simulink library "ddm"  (R2021b)
settings: Solver=VariableStepAuto  StartTime=0.0  StopTime=10.0  RelTol=1e-3
undefined symbols (not defined in the file or in its folder): ENUM_ADASACCSTA_ERROR, ENUM_ADASACCSTA_OFF, ENUM_ADASACCSTA_STANDBY, ENUM_ADASISASTA_OFF, ENUM_ALLOWMOV_ALLOWREADY, ENUM_APS, ENUM_BRKSTA_ERROR, ENUM_BRKSTA_OFF, ENUM_BRKSTA_ON, ENUM_BRKSW_INVALID, ENUM_BRKSW_OFF, ENUM_BRKSW_ON, ENUM_CHGPREACTERRSTA_OBCPRE, ENUM_DCDCFAULTSTA_ANYFAULTLV1, ENUM_DCDCFAULTSTA_ANYFAULTLV2, ENUM_DRIVETRAIN_AWD, ENUM_DRIVETRAIN_FWD, ENUM_DRIVETRAIN_RWD, ENUM_DRSEATSTA_INVALID, ENUM_EDUDRTSTA_NORMAL, ENUM_EPBSTA_APPLIED, ENUM_EPBSTA_RELEASED, ENUM_HVBATTREADYPRE_READY, ENUM_MCUWARN_LV0, ENUM_MCUWARN_LV1, ENUM_MCUWARN_LV2, ENUM_MCUWARN_LV3, ENUM_MCUWARN_NOERROR, ENUM_OBCFAULTSTA_ANYFAULT, ENUM_PAS_R2F2, ENUM_PDFAULT_BATTPDFAIL, ENUM_PDFAULT_DCDCDISABLE, ENUM_PDFAULT_MCUDISABLE, ENUM_PDFAULT_MCUDISCHRG, ENUM_POWERSTA_OFF, ENUM_POWERSTA_ON, ENUM_POWERSTA_READY, ENUM_POWERSTA_STANDBY, ENUM_PRESSINDI_LOW, ENUM_PUFAULT_BATTUPFAIL, ENUM_PUFAULT_DCDCENABLEFAIL, ENUM_PUFAULT_PRECHRGCHKFAIL, ENUM_PUFAULT_SAFETYCHKFAIL, ENUM_PUSTATE_COMPLETED, ENUM_PWRSTASW_OFF, ENUM_PWRSTASW_OFFA, ENUM_PWRSTASW_OFFCHVCHRG, ENUM_PWRSTASW_OFFCLVCHRG, ENUM_PWRSTASW_ON, ENUM_PWRSTASW_ONHVCHRG, ENUM_PWRSTASW_READY, ENUM_PWRSTASW_STANDBY, ENUM_RANGESTA_12IN, ENUM_SHIFTCOMMAND_D, ENUM_SHIFTCOMMAND_N, ENUM_SHIFTCOMMAND_P, ENUM_SHIFTCOMMAND_R, ENUM_VEHMALFUNLV_2ND, ENUM_VEHMALFUNLV_3RD, ENUM_VEHMALFUNLV_4TH ... (+835)
libraries: hcu_lib x750, $bdroot x12, simulink x5
(part 4 of 28)

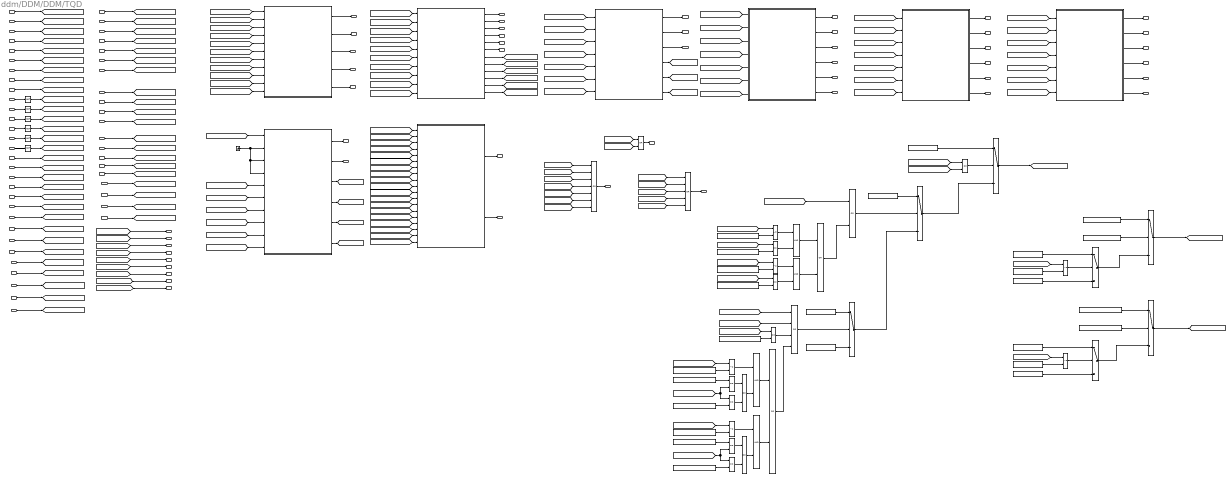
== system ddm/DDM/DDM/TQD ==
  VPMM_SysPwrSta_enum : Inport
  VINP_AccelPedal1Vol_V : Inport  Port=2
  VINP_AccelPedal2Vol_V : Inport  Port=3
  VDHP_EAPS12RangeSta_enum : Inport  Port=4
  VDHP_EAPCRBAD_flg : Inport  Port=5
  task_time_s : Inport  Port=6
  DTC_clear_request : Inport  Port=7
  No_CAN3_BUS_OFF : Inport  Port=8
  No_CAN1_BUS_OFF : Inport  Port=9
  VINP_CANMsgValidMCUF1_flg : Inport  Port=10
  VINP_CANMsgValidMCUR1_flg : Inport  Port=11
  VINP_CANMsgValidShifter1_flg : Inport  Port=12
  VINP_CANMsgValidESC7_flg : Inport  Port=13
  VINP_CANMsgValidESC1_flg : Inport  Port=14
  VINP_CANMsgValidESC5_flg : Inport  Port=15
  VDDM_MCUF1RCErr_flg : Inport  Port=16
  VDDM_MCUF1CSErr_flg : Inport  Port=17
  VDDM_MCUR1RCErr_flg : Inport  Port=18
  VDDM_MCUR1CSErr_flg : Inport  Port=19
  VDDM_Shifter1RCErr_flg : Inport  Port=20
  VDDM_Shifter1CSErr_flg : Inport  Port=21
  VDDM_ESC7RCErr_flg : Inport  Port=22
  VDDM_ESC7CSErr_flg : Inport  Port=23
  VDDM_ESC1RCErr_flg : Inport  Port=24
  VDDM_ESC1CSErr_flg : Inport  Port=25
  VDDM_ESC5RCErr_flg : Inport  Port=26
  VDDM_ESC5CSErr_flg : Inport  Port=27
  VINP_FrEDUDrtSta_flg : Inport  Port=28
  VINP_VehSpeed_kph : Inport  Port=29
  VINP_FrEDURealTMTq_Nm : Inport  Port=30
  VTQR_FrTMTqReq_Nm : Inport  Port=31
  VINP_RrEDUDrtSta_flg : Inport  Port=32
  VINP_RrEDURealTMTq_Nm : Inport  Port=33
  VTQR_RrTMTqReq_Nm : Inport  Port=34
  VINP_MCUWarnF_enum : Inport  Port=35
  VINP_MCUWarnR_enum : Inport  Port=36
  VINP_Pedal1Ref5V_V : Inport  Port=37
  VINP_Pedal2Ref5V_V : Inport  Port=38
  VINP_HVBattSOC_pct : Inport  Port=39
  VDDM_AuxBattVolV_V : Inport  Port=40
  VTQD_ActParkRequest_flg : Inport  Port=41
  VINP_EPBSta_enum : Inport  Port=42
  VINP_ShifterHandleCmd_enum : Inport  Port=43
  VINP_BMSWarn4_flg : Inport  Port=44
  VINP_BMSWarn5_flg : Inport  Port=45
  VINP_BMSWarn6_flg : Inport  Port=46
  VINP_BMSWarn7_flg : Inport  Port=47
  VINP_BMSWarn8_flg : Inport  Port=48
  VINP_DCDCFaultSta_enum : Inport  Port=49
  VPMM_DrivetrainSelect_enum : Inport  Port=50
  APS_DDM : Subsystem
  Constant1 : Constant  Value=ENUM_DRIVETRAIN_FWD
  Constant10 : Constant  Value=ENUM_MCUWARN_LV3
  Constant11 : Constant  Value=ENUM_VEHMALFUNLV_3RD
  Constant12 : Constant  Value=ENUM_VEHMALFUNLV_4TH
  Constant13 : Constant  Value=KDDM_LimpHomeActTmp_flg_ovrdflg  OutDataTypeStr=Inherit: Inherit via back propagation
  Constant14 : Constant  Value=KDDM_LimpHomeActTmp_flg_ovrdval  OutDataTypeStr=Inherit: Inherit via back propagation
  Constant15 : Constant  Value=ENUM_VEHMALFUNLV_2ND
  Constant16 : Constant  Value=ENUM_VEHMALFUNLV_NORMAL
  Constant17 : Constant  Value=ENUM_DCDCFAULTSTA_ANYFAULTLV2
  Constant18 : Constant  Value=ENUM_VEHMALFUNLV_2ND
  Constant19 : Constant  Value=TRUE
  Constant2 : Constant  Value=ENUM_MCUWARN_LV1
  Constant20 : Constant  Value=FALSE
  Constant21 : Constant  Value=ENUM_VEHMALFUNLV_3RD
  Constant22 : Constant  Value=TRUE
  Constant23 : Constant  Value=FALSE
  Constant24 : Constant  Value=KDDM_EDriveSysErrVCUTmp_ovrdflg  OutDataTypeStr=Inherit: Inherit via back propagation
  Constant25 : Constant  Value=KDDM_EDriveSysErrVCUTmp_ovrdval  OutDataTypeStr=Inherit: Inherit via back propagation
  Constant3 : Constant  Value=ENUM_MCUWARN_LV2
  Constant4 : Constant  Value=ENUM_DRIVETRAIN_RWD
  Constant5 : Constant  Value=ENUM_MCUWARN_LV1
  Constant6 : Constant  Value=ENUM_MCUWARN_LV2
  Constant7 : Constant  Value=ENUM_DRIVETRAIN_FWD
  Constant8 : Constant  Value=ENUM_DRIVETRAIN_RWD
  Constant9 : Constant  Value=ENUM_MCUWARN_LV3
  EPB : Subsystem
  ESC1_DDM : Subsystem
  ESC5_DDM : Subsystem
  ESC7_DDM : Subsystem
  Equal{1,5,8,11} (4 alike) : RelationalOperator  Operator=~=  OutDataTypeStr=boolean  RndMeth=Simplest
  Equal{2..4,6..7,9..10} (7 alike) : RelationalOperator  Operator===  OutDataTypeStr=boolean  RndMeth=Simplest
  Equal12 : RelationalOperator  OutDataTypeStr=boolean  RndMeth=Simplest
  Equal13 : RelationalOperator  OutDataTypeStr=boolean  RndMeth=Simplest
  Ground : Ground
  Logical Operator{,1..5} (6 alike) : Logic  Operator=NOT  AllPortsSameDT=off  OutDataTypeStr=boolean
  MCU1_DDM : Subsystem
  MCU_DDM : Subsystem
  OR : Logic  Operator=OR  Inputs=5  AllPortsSameDT=off  OutDataTypeStr=boolean
  OR1 : Logic  Operator=OR  Inputs=7  AllPortsSameDT=off  OutDataTypeStr=boolean
  OR{2,4,6..7,9..10,12} (7 alike) : Logic  Operator=OR  AllPortsSameDT=off  OutDataTypeStr=boolean
  OR{5,8,11,13} (4 alike) : Logic  AllPortsSameDT=off  OutDataTypeStr=boolean
  OR3 : Logic  Operator=OR  Inputs=4  AllPortsSameDT=off  OutDataTypeStr=boolean
  Shifter1_DDM : Subsystem
  Switch{1..7} (7 alike) : Switch  Criteria=u2 ~= 0
  VDDM_APS1SigOoRDTC_raw32 : Outport
  VDDM_APS2SigOoRDTC_raw32 : Outport  Port=2
  VDDM_APSCorrErrDTC_raw32 : Outport  Port=3
  VDDM_MCUF1NoComDTC_raw32 : Outport  Port=4
  VDDM_MCUR1NoComDTC_raw32 : Outport  Port=5
  VDDM_Shifter1NoComDTC_raw32 : Outport  Port=6
  VDDM_ESC7NoComDTC_raw32 : Outport  Port=7
  VDDM_ESC1NoComDTC_raw32 : Outport  Port=8
  VDDM_ESC5NoComDTC_raw32 : Outport  Port=9
  VDDM_MCUF1RCErrDTC_raw32 : Outport  Port=10
  VDDM_MCUR1RCErrDTC_raw32 : Outport  Port=11
  VDDM_MCUF1CSErrDTC_raw32 : Outport  Port=12
  VDDM_MCUR1CSErrDTC_raw32 : Outport  Port=13
  VDDM_Shifter1RCErrDTC_raw32 : Outport  Port=14
  VDDM_Shifter1CSErrDTC_raw32 : Outport  Port=15
  VDDM_ESC7RCErrDTC_raw32 : Outport  Port=16
  VDDM_ESC7CSErrDTC_raw32 : Outport  Port=17
  VDDM_ESC1RCErrDTC_raw32 : Outport  Port=18
  VDDM_ESC1CSErrDTC_raw32 : Outport  Port=19
  VDDM_ESC5RCErrDTC_raw32 : Outport  Port=20
  VDDM_ESC5CSErrDTC_raw32 : Outport  Port=21
  VDDM_FrMCUTqErrDTC_raw32 : Outport  Port=22
  VDDM_RrMCUTqErrDTC_raw32 : Outport  Port=23
  VDDM_MCUF1NoComCFS_flg : Outport  Port=24
  VDDM_MCUF1RCErrCFS_flg : Outport  Port=25
  VDDM_MCUF1CSErrCFS_flg : Outport  Port=26
  VDDM_MCUR1NoComCFS_flg : Outport  Port=27
  VDDM_MCUR1RCErrCFS_flg : Outport  Port=28
  VDDM_MCUR1CSErrCFS_flg : Outport  Port=29
  VDDM_ESC7NoComCFS_flg : Outport  Port=30
  VDDM_ESC7RCErrCFS_flg : Outport  Port=31
  VDDM_ESC7CSErrCFS_flg : Outport  Port=32
  VDDM_ESC1NoComCFS_flg : Outport  Port=33
  VDDM_ESC1RCErrCFS_flg : Outport  Port=34
  VDDM_ESC1CSErrCFS_flg : Outport  Port=35
  VDDM_ESC5NoComCFS_flg : Outport  Port=36
  VDDM_ESC5RCErrCFS_flg : Outport  Port=37
  VDDM_ESC5CSErrCFS_flg : Outport  Port=38
  VDDM_5vAPS1PwrErrDTC_raw32 : Outport  Port=39
  VDDM_5vAPS2PwrErrDTC_raw32 : Outport  Port=40
  VDDM_EPBLockTODTC_raw32 : Outport  Port=41
  VDDM_EPBUnlockTODTC_raw32 : Outport  Port=42
  EDriveSysErr_VCUErr : Outport  Port=43
  EDriveSysErr_ShifterErr : Outport  Port=44
  EngageP_Fail : Outport  Port=45
  VDDM_LimpHomeActTmp_flg : Outport  Port=46
  VDDM_EDriveSysErr_VCUErrTmp_flg : Outport  Port=47
  VDDM_VehMalfunLevelTmp_enum : Outport  Port=48
  wires:
  VINP_ShifterHandleCmd_enum/1 -> [VINP_ShifterHandleCmd_enum]
  VINP_EPBSta_enum/1 -> [VINP_EPBSta_enum]
  VTQD_ActParkRequest_flg/1 -> [VTQD_ActParkRequest_flg]
  EPB/2(VDDM_EPBUnlockTODTC_raw32) -> VDDM_EPBUnlockTODTC_raw32/1
  EPB/1(VDDM_EPBLockTODTC_raw32) -> VDDM_EPBLockTODTC_raw32/1
  [VINP_EPBSta_enum] -> EPB/7(VINP_EPBSta_enum)
  [VTQD_ActParkRequest_flg] -> EPB/6(VTQD_ActParkRequest_flg)
  [VINP_ShifterHandleCmd_enum] -> EPB/8(VINP_ShifterHandleCmd_enum)
  [VPMM_SysPwrSta_enum] -> EPB/5(VPMM_SysPwrSta_enum)
  [task_time_s] -> EPB/9(task_time_s)
  [No_CAN1_BUS_OFF] -> EPB/1(NO_CAN1_BUS_OFF)
  [DTC_clear_request] -> EPB/10(DTC_clear_request)
  Ground/1 -> EPB/2(CAN_LossOfEPB1), EPB/3(RC_LossErrOfEPB1), EPB/4(CS_LossErrOfEPB1)
  [VDDM_AuxBattVolV_V] -> APS_DDM/11(VDDM_AuxBattVolV_V)
  VDDM_AuxBattVolV_V/1 -> [VDDM_AuxBattVolV_V]
  APS_DDM/5(VDDM_5vAPS2PwrErrDTC_raw32) -> VDDM_5vAPS2PwrErrDTC_raw32/1
  APS_DDM/4(VDDM_5vAPS1PwrErrDTC_raw32) -> VDDM_5vAPS1PwrErrDTC_raw32/1
  [VINP_HVBattSOC_pct] -> APS_DDM/8(VINP_HVBattSOC_pct)
  VINP_HVBattSOC_pct/1 -> [VINP_HVBattSOC_pct]
  [VINP_Pedal2Ref5V_V] -> APS_DDM/7(VINP_Pedal2Ref5V_V)
  [VINP_Pedal1Ref5V_V] -> APS_DDM/6(VINP_Pedal1Ref5V_V)
  VINP_Pedal2Ref5V_V/1 -> [VINP_Pedal2Ref5V_V]
  VINP_Pedal1Ref5V_V/1 -> [VINP_Pedal1Ref5V_V]
  [VDDM_MCUR1RCErrCFS_flg] -> MCU_DDM/12(VDDM_MCUR1RCErrCFS_flg)
  [VDDM_MCUF1RCErrCFS_flg] -> MCU_DDM/5(VDDM_MCUF1RCErrCFS_flg)
  [VDDM_MCUF1CSErrCFS_flg] -> MCU_DDM/6(VDDM_MCUF1CSErrCFS_flg)
  [No_CAN3_BUS_OFF] -> MCU_DDM/3(No_CAN3_BUS_OFF)
  [VINP_MCUWarnF_enum] -> MCU_DDM/17(VINP_MCUWarnF_enum)
  [VINP_RrEDUDrtSta_flg] -> MCU_DDM/14(VINP_RrEDUDrtSta_flg)
  [VDDM_MCUR1CSErrCFS_flg] -> MCU_DDM/13(VDDM_MCUR1CSErrCFS_flg)
  [VPMM_SysPwrSta_enum] -> MCU_DDM/2(VPMM_SysPwrSta_enum)
  [VDDM_MCUF1NoComCFS_flg] -> MCU_DDM/4(VDDM_MCUF1NoComCFS_flg)
  [VTQR_FrTMTqReq_Nm] -> MCU_DDM/10(VTQR_FrTMTqReq_Nm)
  [task_time_s] -> MCU_DDM/1(task_time_s)
  [VTQR_RrTMTqReq_Nm] -> MCU_DDM/16(VTQR_RrTMTqReq_Nm)
  [VINP_FrEDUDrtSta_flg] -> MCU_DDM/8(VINP_FrEDUDrtSta_flg)
  [VINP_FrEDURealTMTq_Nm] -> MCU_DDM/9(VINP_FrEDURealTMTq_Nm)
  [VINP_RrEDURealTMTq_Nm] -> MCU_DDM/15(VINP_RrEDURealTMTq_Nm)
  [DTC_clear_request] -> MCU_DDM/19(DTC_clear_request)
  [VDDM_MCUR1NoComCFS_flg] -> MCU_DDM/11(VDDM_MCUR1NoComCFS_flg)
  [VINP_MCUWarnR_enum] -> MCU_DDM/18(VINP_MCUWarnR_enum)
  [VINP_VehSpeed_kph] -> MCU_DDM/7(VINP_VehSpeed_kph)
  [VDDM_MCUF1RCErrCFS_flg] -> VDDM_MCUF1RCErrCFS_flg/1
  [VDDM_MCUR1RCErrCFS_flg] -> VDDM_MCUR1RCErrCFS_flg/1
  [VDDM_MCUR1NoComCFS_flg] -> VDDM_MCUR1NoComCFS_flg/1
  [VDDM_MCUF1CSErrCFS_flg] -> VDDM_MCUF1CSErrCFS_flg/1
  [VDDM_MCUR1CSErrCFS_flg] -> VDDM_MCUR1CSErrCFS_flg/1
  [VDDM_MCUF1NoComCFS_flg] -> VDDM_MCUF1NoComCFS_flg/1
  MCU1_DDM/11(VDDM_MCUR1RCErrCFS_flg) -> [VDDM_MCUR1RCErrCFS_flg]
  MCU1_DDM/7(VDDM_MCUF1NoComCFS_flg) -> [VDDM_MCUF1NoComCFS_flg]
  MCU1_DDM/10(VDDM_MCUR1NoComCFS_flg) -> [VDDM_MCUR1NoComCFS_flg]
  MCU1_DDM/9(VDDM_MCUF1CSErrCFS_flg) -> [VDDM_MCUF1CSErrCFS_flg]
  MCU1_DDM/8(VDDM_MCUF1RCErrCFS_flg) -> [VDDM_MCUF1RCErrCFS_flg]
  MCU1_DDM/12(VDDM_MCUR1CSErrCFS_flg) -> [VDDM_MCUR1CSErrCFS_flg]
  VINP_MCUWarnR_enum/1 -> [VINP_MCUWarnR_enum]
  VINP_MCUWarnF_enum/1 -> [VINP_MCUWarnF_enum]
  ESC1_DDM/6(VDDM_ESC1CSErrCFS_flg) -> VDDM_ESC1CSErrCFS_flg/1
  ESC1_DDM/4(VDDM_ESC1NoComCFS_flg) -> VDDM_ESC1NoComCFS_flg/1
  ESC5_DDM/5(VDDM_ESC5RCErrCFS_flg) -> VDDM_ESC5RCErrCFS_flg/1
  ESC1_DDM/5(VDDM_ESC1RCErrCFS_flg) -> VDDM_ESC1RCErrCFS_flg/1
  ESC5_DDM/4(VDDM_ESC5NoComCFS_flg) -> VDDM_ESC5NoComCFS_flg/1
  ESC5_DDM/6(VDDM_ESC5CSErrCFS_flg) -> VDDM_ESC5CSErrCFS_flg/1
  ESC7_DDM/4(VDDM_ESC7NoComCFS_flg) -> VDDM_ESC7NoComCFS_flg/1
  ESC7_DDM/5(VDDM_ESC7RCErrCFS_flg) -> VDDM_ESC7RCErrCFS_flg/1
  ESC7_DDM/6(VDDM_ESC7CSErrCFS_flg) -> VDDM_ESC7CSErrCFS_flg/1
  VINP_VehSpeed_kph/1 -> [VINP_VehSpeed_kph]
  VINP_RrEDUDrtSta_flg/1 -> [VINP_RrEDUDrtSta_flg]
  VTQR_FrTMTqReq_Nm/1 -> [VTQR_FrTMTqReq_Nm]
  VINP_FrEDURealTMTq_Nm/1 -> [VINP_FrEDURealTMTq_Nm]
  VTQR_RrTMTqReq_Nm/1 -> [VTQR_RrTMTqReq_Nm]
  VINP_FrEDUDrtSta_flg/1 -> [VINP_FrEDUDrtSta_flg]
  VINP_RrEDURealTMTq_Nm/1 -> [VINP_RrEDURealTMTq_Nm]
  VDDM_ESC5RCErr_flg/1 -> [VDDM_ESC5RCErr_flg]
  VDDM_ESC5CSErr_flg/1 -> [VDDM_ESC5CSErr_flg]
  [VDDM_ESC5CSErr_flg] -> ESC5_DDM/6(VDDM_ESC5CSErr_flg)
  [VDDM_ESC5RCErr_flg] -> ESC5_DDM/5(VDDM_ESC5RCErr_flg)
  VDDM_ESC1RCErr_flg/1 -> [VDDM_ESC1RCErr_flg]
  VDDM_ESC1CSErr_flg/1 -> [VDDM_ESC1CSErr_flg]
  [VDDM_ESC1CSErr_flg] -> ESC1_DDM/6(VDDM_ESC1CSErr_flg)
  [VDDM_ESC1RCErr_flg] -> ESC1_DDM/5(VDDM_ESC1RCErr_flg)
  VDDM_ESC7RCErr_flg/1 -> [VDDM_ESC7RCErr_flg]
  VDDM_ESC7CSErr_flg/1 -> [VDDM_ESC7CSErr_flg]
  [VDDM_ESC7CSErr_flg] -> ESC7_DDM/6(VDDM_ESC7CSErr_flg)
  [VDDM_ESC7RCErr_flg] -> ESC7_DDM/5(VDDM_ESC7RCErr_flg)
  VDDM_Shifter1CSErr_flg/1 -> [VDDM_Shifter1CSErr_flg]
  VDDM_Shifter1RCErr_flg/1 -> [VDDM_Shifter1RCErr_flg]
  VDDM_MCUF1RCErr_flg/1 -> [VDDM_MCUF1RCErr_flg]
  VDDM_MCUF1CSErr_flg/1 -> [VDDM_MCUF1CSErr_flg]
  VDDM_MCUR1CSErr_flg/1 -> [VDDM_MCUR1CSErr_flg]
  VDDM_MCUR1RCErr_flg/1 -> [VDDM_MCUR1RCErr_flg]
  [VDDM_Shifter1CSErr_flg] -> Shifter1_DDM/6(VDDM_Shifter1CSErr_flg)
  [VDDM_Shifter1RCErr_flg] -> Shifter1_DDM/5(VDDM_Shifter1RCErr_flg)
  MCU_DDM/1(VDDM_FrMCUTqErrDTC_raw32) -> VDDM_FrMCUTqErrDTC_raw32/1
  MCU_DDM/2(VDDM_RrMCUTqErrDTC_raw32) -> VDDM_RrMCUTqErrDTC_raw32/1
  ESC5_DDM/3(VDDM_ESC5CSErrDTC_raw32) -> VDDM_ESC5CSErrDTC_raw32/1
  ESC5_DDM/2(VDDM_ESC5RCErrDTC_raw32) -> VDDM_ESC5RCErrDTC_raw32/1
  ESC1_DDM/2(VDDM_ESC1RCErrDTC_raw32) -> VDDM_ESC1RCErrDTC_raw32/1
  ESC1_DDM/3(VDDM_ESC1CSErrDTC_raw32) -> VDDM_ESC1CSErrDTC_raw32/1
  ESC7_DDM/3(VDDM_ESC7CSErrDTC_raw32) -> VDDM_ESC7CSErrDTC_raw32/1
  ESC7_DDM/2(VDDM_ESC7RCErrDTC_raw32) -> VDDM_ESC7RCErrDTC_raw32/1
  Shifter1_DDM/3(VDDM_Shifter1CSErrDTC_raw32) -> VDDM_Shifter1CSErrDTC_raw32/1
  Shifter1_DDM/2(VDDM_Shifter1RCErrDTC_raw32) -> VDDM_Shifter1RCErrDTC_raw32/1
  MCU1_DDM/6(VDDM_MCUR1CSErrDTC_raw32) -> VDDM_MCUR1CSErrDTC_raw32/1
  MCU1_DDM/5(VDDM_MCUF1CSErrDTC_raw32) -> VDDM_MCUF1CSErrDTC_raw32/1
  MCU1_DDM/3(VDDM_MCUF1RCErrDTC_raw32) -> VDDM_MCUF1RCErrDTC_raw32/1
  MCU1_DDM/4(VDDM_MCUR1RCErrDTC_raw32) -> VDDM_MCUR1RCErrDTC_raw32/1
  ESC7_DDM/1(VDDM_ESC7NoComDTC_raw32) -> VDDM_ESC7NoComDTC_raw32/1
  [VDDM_MCUR1CSErr_flg] -> MCU1_DDM/9(VDDM_MCUR1CSErr_flg)
  [VDDM_MCUR1RCErr_flg] -> MCU1_DDM/8(VDDM_MCUR1RCErr_flg)
  [VDDM_MCUF1CSErr_flg] -> MCU1_DDM/7(VDDM_MCUF1CSErr_flg)
  [VDDM_MCUF1RCErr_flg] -> MCU1_DDM/6(VDDM_MCUF1RCErr_flg)
  Logical Operator5/1 -> [VDDM_MCUF1NoCom_flg]
  Logical Operator4/1 -> [VDDM_MCUR1NoCom_flg]
  Logical Operator3/1 -> [VDDM_Shifter1NoCom_flg]
  Logical Operator2/1 -> [VDDM_ESC7NoCom_flg]
  Logical Operator1/1 -> [VDDM_ESC1NoCom_flg]
  Logical Operator/1 -> [VDDM_ESC5NoCom_flg]
  VINP_CANMsgValidESC5_flg/1 -> Logical Operator/1
  VINP_CANMsgValidESC1_flg/1 -> Logical Operator1/1
  VINP_CANMsgValidESC7_flg/1 -> Logical Operator2/1
  VINP_CANMsgValidShifter1_flg/1 -> Logical Operator3/1
  VINP_CANMsgValidMCUR1_flg/1 -> Logical Operator4/1
  VINP_CANMsgValidMCUF1_flg/1 -> Logical Operator5/1
  No_CAN1_BUS_OFF/1 -> [No_CAN1_BUS_OFF]
  No_CAN3_BUS_OFF/1 -> [No_CAN3_BUS_OFF]
  ESC5_DDM/1(VDDM_ESC5NoComDTC_raw32) -> VDDM_ESC5NoComDTC_raw32/1
  ESC1_DDM/1(VDDM_ESC1NoComDTC_raw32) -> VDDM_ESC1NoComDTC_raw32/1
  Shifter1_DDM/1(VDDM_Shifter1NoComDTC_raw32) -> VDDM_Shifter1NoComDTC_raw32/1
  MCU1_DDM/2(VDDM_MCUR1NoComDTC_raw32) -> VDDM_MCUR1NoComDTC_raw32/1
  MCU1_DDM/1(VDDM_MCUF1NoComDTC_raw32) -> VDDM_MCUF1NoComDTC_raw32/1
  [DTC_clear_request] -> ESC5_DDM/7(DTC_clear_request)
  [VDDM_ESC5NoCom_flg] -> ESC5_DDM/4(VDDM_ESC5NoCom_flg)
  [No_CAN1_BUS_OFF] -> ESC5_DDM/3(No_CAN1_BUS_OFF)
  [VPMM_SysPwrSta_enum] -> ESC5_DDM/2(VPMM_SysPwrSta_enum)
  [task_time_s] -> ESC5_DDM/1(task_time_s)
  [DTC_clear_request] -> ESC1_DDM/7(DTC_clear_request)
  [VDDM_ESC1NoCom_flg] -> ESC1_DDM/4(VDDM_ESC1NoCom_flg)
  [No_CAN1_BUS_OFF] -> ESC1_DDM/3(No_CAN1_BUS_OFF)
  [VPMM_SysPwrSta_enum] -> ESC1_DDM/2(VPMM_SysPwrSta_enum)
  [task_time_s] -> ESC1_DDM/1(task_time_s)
  [DTC_clear_request] -> ESC7_DDM/7(DTC_clear_request)
  [VPMM_SysPwrSta_enum] -> ESC7_DDM/2(VPMM_SysPwrSta_enum)
  [No_CAN1_BUS_OFF] -> ESC7_DDM/3(No_CAN1_BUS_OFF)
  [VDDM_ESC7NoCom_flg] -> ESC7_DDM/4(VDDM_ESC7NoCom_flg)
  [DTC_clear_request] -> Shifter1_DDM/7(DTC_clear_request)
  [VDDM_Shifter1NoCom_flg] -> Shifter1_DDM/4(VDDM_Shifter1NoCom_flg)
  [No_CAN3_BUS_OFF] -> Shifter1_DDM/3(No_CAN3_BUS_OFF)
  [VPMM_SysPwrSta_enum] -> Shifter1_DDM/2(VPMM_SysPwrSta_enum)
  [DTC_clear_request] -> MCU1_DDM/10(DTC_clear_request)
  [VDDM_MCUR1NoCom_flg] -> MCU1_DDM/5(VDDM_MCUR1NoCom_flg)
  [VDDM_MCUF1NoCom_flg] -> MCU1_DDM/4(VDDM_MCUF1NoCom_flg)
  [No_CAN3_BUS_OFF] -> MCU1_DDM/3(No_CAN3_BUS_OFF)
  [VPMM_SysPwrSta_enum] -> MCU1_DDM/2(VPMM_SysPwrSta_enum)
  [task_time_s] -> ESC7_DDM/1(task_time_s)
  [task_time_s] -> Shifter1_DDM/1(task_time_s)
  [task_time_s] -> MCU1_DDM/1(task_time_s)
  [DTC_clear_request] -> APS_DDM/10(DTC_clear_request)
  DTC_clear_request/1 -> [DTC_clear_request]
  [task_time_s] -> APS_DDM/9(task_time_s)
  task_time_s/1 -> [task_time_s]
  APS_DDM/3(VDDM_APSCorrErrDTC_raw32) -> VDDM_APSCorrErrDTC_raw32/1
  APS_DDM/2(VDDM_APS2SigOoRDTC_raw32) -> VDDM_APS2SigOoRDTC_raw32/1
  APS_DDM/1(VDDM_APS1SigOoRDTC_raw32) -> VDDM_APS1SigOoRDTC_raw32/1
  [VDHP_EAPS12RangeSta_enum] -> APS_DDM/4(VDHP_EAPS12RangeSta_enum)
  [VINP_AccelPedal2Vol_V] -> APS_DDM/3(VINP_AccelPedal2Vol_V)
  [VINP_AccelPedal1Vol_V] -> APS_DDM/2(VINP_AccelPedal1Vol_V)
  [VPMM_SysPwrSta_enum] -> APS_DDM/1(VPMM_SysPwrSta_enum)
  [VDHP_EAPCRBAD_flg] -> APS_DDM/5(VDHP_EAPCRBAD_flg)
  VPMM_SysPwrSta_enum/1 -> [VPMM_SysPwrSta_enum]
  VINP_AccelPedal1Vol_V/1 -> [VINP_AccelPedal1Vol_V]
  VDHP_EAPCRBAD_flg/1 -> [VDHP_EAPCRBAD_flg]
  VDHP_EAPS12RangeSta_enum/1 -> [VDHP_EAPS12RangeSta_enum]
  VINP_AccelPedal2Vol_V/1 -> [VINP_AccelPedal2Vol_V]
  EPB/3(VDDM_EPBLockTODFS_flg) -> [VDDM_EPBLockTODFS_flg]
  EPB/4(VDDM_EPBLockTOCFS_flg) -> [VDDM_EPBLockTOCFS_flg]
  EPB/5(VDDM_EPBUnlockTODFS_flg) -> [VDDM_EPBUnlockTODFS_flg]
  EPB/6(VDDM_EPBUnlockTOCFS_flg) -> [VDDM_EPBUnlockTOCFS_flg]
  Shifter1_DDM/4(VDDM_Shifter1NoComCFS_flg) -> [VDDM_Shifter1NoComCFS_flg]
  Shifter1_DDM/5(VDDM_Shifter1RCErrCFS_flg) -> [VDDM_Shifter1RCErrCFS_flg]
  Shifter1_DDM/6(VDDM_Shifter1CSErrCFS_flg) -> [VDDM_Shifter1CSErrCFS_flg]
  OR/1 -> EDriveSysErr_VCUErr/1
  OR1/1 -> EDriveSysErr_ShifterErr/1
  [VDDM_Shifter1RCErrCFS_flg] -> OR1/2
  [VDDM_Shifter1NoComCFS_flg] -> OR1/1
  [VDDM_Shifter1CSErrCFS_flg] -> OR1/3
  [VDDM_EPBLockTODFS_flg] -> OR1/4
  [VDDM_EPBLockTOCFS_flg] -> OR1/5
  [VDDM_EPBUnlockTODFS_flg] -> OR1/6
  [VDDM_EPBUnlockTOCFS_flg] -> OR1/7
  [VDDM_Shifter1RCErrCFS_flg] -> OR/2
  [VDDM_Shifter1CSErrCFS_flg] -> OR/3
  [VDDM_Shifter1NoComCFS_flg] -> OR/1
  [VDDM_EPBLockTOCFS_flg] -> OR/4
  [VDDM_EPBUnlockTOCFS_flg] -> OR/5
  OR2/1 -> EngageP_Fail/1
  [VDDM_EPBUnlockTOCFS_flg] -> OR2/1
  [VDDM_EPBLockTOCFS_flg] -> OR2/2
  VINP_BMSWarn4_flg/1 -> [VINP_BMSWarn4_flg]
  VINP_BMSWarn5_flg/1 -> [VINP_BMSWarn5_flg]
  VINP_BMSWarn6_flg/1 -> [VINP_BMSWarn6_flg]
  VINP_BMSWarn7_flg/1 -> [VINP_BMSWarn7_flg]
  VINP_BMSWarn8_flg/1 -> [VINP_BMSWarn8_flg]
  VINP_DCDCFaultSta_enum/1 -> [VINP_DCDCFaultSta_enum]
  [VINP_BMSWarn4_flg] -> OR3/1
  [VINP_BMSWarn5_flg] -> OR3/2
  OR3/1 -> Switch6/2
  Constant15/1 -> Switch6/1
  [VINP_BMSWarn7_flg] -> OR4/1
  [VINP_BMSWarn8_flg] -> OR4/2
  Constant17/1 -> Equal2/2
  [VINP_DCDCFaultSta_enum] -> Equal2/1
  Equal2/1 -> OR3/3
  VPMM_DrivetrainSelect_enum/1 -> [VPMM_DrivetrainSelect_enum]
  [VPMM_DrivetrainSelect_enum] -> Equal1/1
  Constant1/1 -> Equal1/2
  Equal1/1 -> OR5/1
  [VINP_MCUWarnR_enum] -> Equal4/1, Equal3/2
  Constant2/1 -> Equal3/1
  Equal3/1 -> OR6/1
  Constant3/1 -> Equal4/2
  Equal4/1 -> OR6/2
  OR6/1 -> OR5/2
  OR5/1 -> OR7/1
  OR7/1 -> OR3/4
  Constant5/1 -> Equal6/1
  Equal7/1 -> OR9/2
  Constant6/1 -> Equal7/2
  Equal6/1 -> OR9/1
  [VINP_MCUWarnF_enum] -> Equal7/1, Equal6/2
  [VPMM_DrivetrainSelect_enum] -> Equal5/1
  OR9/1 -> OR8/2
  Constant4/1 -> Equal5/2
  Equal5/1 -> OR8/1
  OR8/1 -> OR7/2
  [VINP_BMSWarn6_flg] -> OR10/1
  Equal10/1 -> OR11/2
  Constant9/1 -> Equal10/2
  [VINP_MCUWarnR_enum] -> Equal10/1
  [VPMM_DrivetrainSelect_enum] -> Equal8/1
  Constant7/1 -> Equal8/2
  Equal8/1 -> OR11/1
  OR11/1 -> OR12/1
  Constant8/1 -> Equal11/2
  Equal11/1 -> OR13/1
  [VPMM_DrivetrainSelect_enum] -> Equal11/1
  Constant10/1 -> Equal9/2
  [VINP_MCUWarnF_enum] -> Equal9/1
  Equal9/1 -> OR13/2
  OR13/1 -> OR12/2
  OR12/1 -> OR10/2
  OR4/1 -> Switch1/2
  Constant12/1 -> Switch1/1
  Switch1/1 -> [VDDM_VehMalfunLevelTmp_enum]  "VDDM_VehMalfunLevelTmp_enum"
  OR10/1 -> Switch2/2
  Constant11/1 -> Switch2/1
  Switch2/1 -> Switch1/3
  Switch6/1 -> Switch2/3
  Constant16/1 -> Switch6/3
  Constant13/1 -> Switch3/2
  Constant14/1 -> Switch3/1
  [VDDM_VehMalfunLevelTmp_enum] -> Equal12/1
  Switch3/1 -> [VDDM_LimpHomeActTmp_flg]  "VDDM_LimpHomeActTmp_flg"
  Constant18/1 -> Equal12/2
  Equal12/1 -> Switch4/2
  Constant19/1 -> Switch4/1
  Constant20/1 -> Switch4/3
  Switch4/1 -> Switch3/3
  [VDDM_LimpHomeActTmp_flg] -> VDDM_LimpHomeActTmp_flg/1
  Constant22/1 -> Switch5/1
  Constant23/1 -> Switch5/3
  Equal13/1 -> Switch5/2
  Constant21/1 -> Equal13/2
  [VDDM_VehMalfunLevelTmp_enum] -> Equal13/1
  Switch5/1 -> Switch7/3
  Constant25/1 -> Switch7/1
  Constant24/1 -> Switch7/2
  Switch7/1 -> [VDDM_EDriveSysErr_VCUErrTmp_flg]  "VDDM_EDriveSysErr_VCUErrTmp_flg"
  [VDDM_EDriveSysErr_VCUErrTmp_flg] -> VDDM_EDriveSysErr_VCUErrTmp_flg/1
  [VDDM_VehMalfunLevelTmp_enum] -> VDDM_VehMalfunLevelTmp_enum/1
